simulink model "Heat_Exchanger_v2"  (R2020b)
settings: Solver=ode4  StartTime=0.0  StopTime=1000.0  FixedStep=0.01  RelTol=1e-3
values from neighbouring files (symbols this model uses):
  At = nt .* 2 .* pi .* D_t .* dL    [parat_heat_exchanger.m]
  C_w = 490    [parat_heat_exchanger.m]
  Cp_c = 4005    [parat_heat_exchanger.m]
  Cp_h = 4187    [parat_heat_exchanger.m]
  dt = 0.01    [parat_heat_exchanger.m]
  HTC_ref = 350    [parat_heat_exchanger.m]
  m_ref = 3.5    [parat_heat_exchanger.m]
  mass_c = density_c * Ac * dL    [parat_heat_exchanger.m]
  mass_h = density_h * Ah * dL    [parat_heat_exchanger.m]
  mass_w = density_w * Aw * dL    [parat_heat_exchanger.m]
  mh_start = 2.5    [parat_heat_exchanger.m]
  N = 100    [parat_heat_exchanger.m]
  Tcin = 289    [parat_heat_exchanger.m]
  Tenv = 295    [parat_heat_exchanger.m]
  Thin = 363    [parat_heat_exchanger.m]
  Tref = 348    [parat_heat_exchanger.m]
undefined symbols (not defined in the file or in its folder): Tc_init, Th_init, Tw_init
libraries: pid_lib x1
settings Model: Creator=kzlsahin  LastModifiedBy=kzlsahin

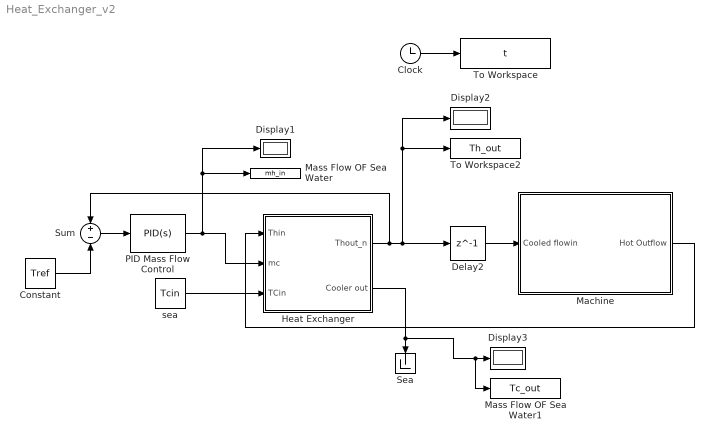
== system Heat_Exchanger_v2 ==
  Clock : Clock
  Constant : Constant  Value=Tref
  Delay2 : Delay  DelayLength=1  InitialCondition=Tenv
  Display1 : Display
  Display2 : Display
  Display3 : Display
  Heat Exchanger : Subsystem
      mask Display: image('/home/kzlsahin/Documents/yüksek lisans/MTME/ödev/iconHXtrans.jpeg'); % Use "Edit Image" on toolstrip to change.
  Machine : Subsystem
  Mass Flow OF Sea Water : ToWorkspace  VariableName=mh_in  SampleTime=-1
  Mass Flow OF Sea Water1 : ToWorkspace  VariableName=Tc_out  SampleTime=-1
  PID Mass Flow Control : pid_lib/PID Controller  Controller=PID  Form=Parallel  TimeDomain=Continuous-time  UseExternalTs=on  SampleTime=-1  IntegratorMethod=Forward Euler  FilterMethod=Forward Euler  ControllerParametersSource=internal  P=1  I=1  D=1  UseFilter=on  N=100  TunerSelectOption=Transfer Function Based (PID Tuner App)  InitialConditionSource=internal  InitialConditionForIntegrator=0  InitialConditionForFilter=0  DifferentiatorICPrevScaledInput=0  ExternalReset=none  TrackingMode=off  Kt=1  LimitOutput=on  SatLimitsSource=internal  UpperSaturationLimit=10  LowerSaturationLimit=0.5  LinearizeAsGain=on  AntiWindupMode=none  Kb=1  POutMin=[]  POutMax=[]  IOutMin=[]  IOutMax=[]  DOutMin=[]  DOutMax=[]  NOutMin=[]  NOutMax=[]  SumOutMin=[]  SumOutMax=[]  SaturationOutMin=[]  SaturationOutMax=[]  PParamMin=[]  PParamMax=[]  IParamMin=[]  IParamMax=[]  DParamMin=[]  DParamMax=[]  NParamMin=[]  NParamMax=[]  KbParamMin=[]  KbParamMax=[]  KtParamMin=[]  KtParamMax=[]  KbOutMin=[]  KbOutMax=[]  KtOutMin=[]  KtOutMax=[]  IntegratorOutMin=[]  IntegratorOutMax=[]  FilterOutMin=[]  FilterOutMax=[]  SumI1OutMin=[]  SumI1OutMax=[]  SumI2OutMin=[]  SumI2OutMax=[]  SumI3OutMin=[]  SumI3OutMax=[]  SumI4OutMin=[]  SumI4OutMax=[]  SumDOutMin=[]  SumDOutMax=[]  DifferentiatorOutMin=[]  DifferentiatorOutMax=[]  FilterDiffOutCoefMin=[]  FilterDiffOutCoefMax=[]  ReciprocalOutMin=[]  ReciprocalOutMax=[]  SumDenOutMin=[]  SumDenOutMax=[]  SumNumOutMin=[]  SumNumOutMax=[]  DivideOutMin=[]  DivideOutMax=[]  UdiffTsProdOutMin=[]  UdiffTsProdOutMax=[]  NTsProdOutMin=[]  NTsProdOutMax=[]  UintegralTsProdOutMin=[]  UintegralTsProdOutMax=[]  UngainTsProdOutMin=[]  UngainTsProdOutMax=[]  IntegratorContinuousStateAttributes=''  IntegratorStateMustResolveToSignalObject=off  IntegratorRTWStateStorageClass=Auto  FilterContinuousStateAttributes=''  FilterStateMustResolveToSignalObject=off  FilterRTWStateStorageClass=Auto  ParallelPVariant=InternalParameters  IdealPVariant=Disabled  IVariant=InternalParameters  DVariant=InternalParameters  IntegratorVariant=Continuous  SatVariant=Enabled  AWVariant=Passthrough  PCopyVariant=Disabled  TRVariant=Disabled  FdbkBlocksVariant=Forward  IdealPFdbkVariant=Disabled  SatFdbkVariant=Disabled  DerivativeFilterVariant=ContFilter  NVariant=InternalParameters  NCopyVariant=Disabled  FilterICVariant=InternalICsFilter  IntegratorICVariant=InternalICs  ExternalResetVariant=Disabled  TRSumVariant=Passthrough  SumFdbkVariant=Disabled  SumVariant=Sum_PID  TsampFilterVariant=InternalTs  TsampNgainVariant=Passthrough  TsampIntegralVariant=Passthrough  ExternalSaturationOutDataTypeStr=Inherit: Same as second input
  Sea : Terminator
  Sum : Sum  Inputs=+-
  To Workspace : ToWorkspace  VariableName=t  SampleTime=-1
  To Workspace2 : ToWorkspace  VariableName=Th_out  SampleTime=-1
  sea : Constant  Value=Tcin
  wires:
  Sum/1 -> PID Mass Flow Control/1
  Machine/1(Hot Outflow) -> Heat Exchanger/1(Thin)
  Clock/1 -> To Workspace/1
  Heat Exchanger/1(Thout_n) -> Display2/1, To Workspace2/1, Delay2/1, Sum/1
  Delay2/1 -> Machine/1(Cooled flowin)
  Heat Exchanger/2(Cooler out) -> Mass Flow OF Sea Water1/1, Display3/1, Sea/1
  sea/1 -> Heat Exchanger/3(TCin)
  PID Mass Flow Control/1 -> Heat Exchanger/2(mc), Display1/1, Mass Flow OF Sea Water/1
  Constant/1 -> Sum/2

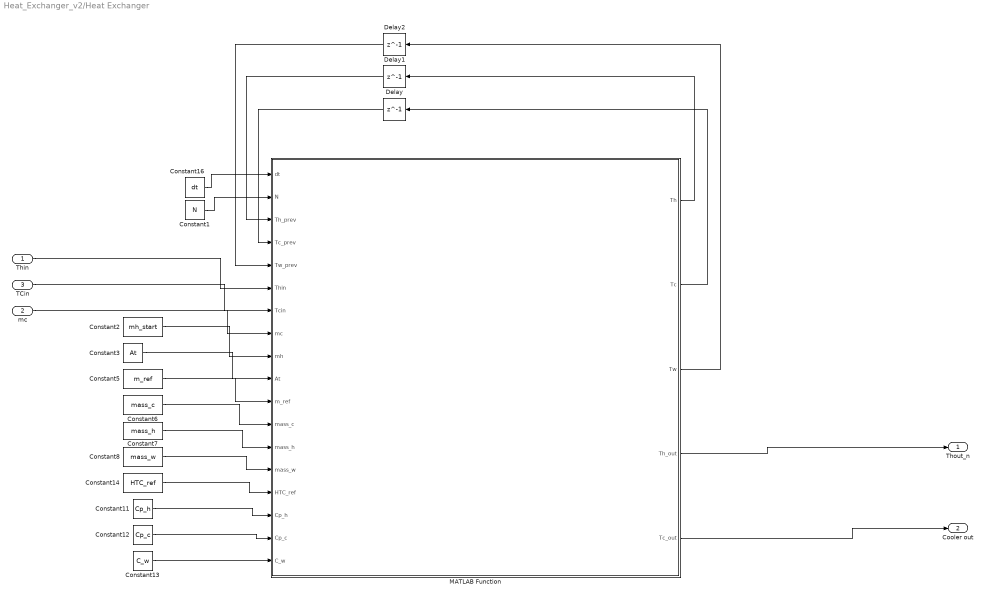
== system Heat_Exchanger_v2/Heat Exchanger ==
  Thin : Inport
  mc : Inport  Port=2
  TCin : Inport  Port=3
  Constant1 : Constant  Value=N
  Constant11 : Constant  Value=Cp_h
  Constant12 : Constant  Value=Cp_c
  Constant13 : Constant  Value=C_w
  Constant14 : Constant  Value=HTC_ref
  Constant16 : Constant  Value=dt
  Constant2 : Constant  Value=mh_start
  Constant3 : Constant  Value=At
  Constant5 : Constant  Value=m_ref
  Constant6 : Constant  Value=mass_c
  Constant7 : Constant  Value=mass_h
  Constant8 : Constant  Value=mass_w
  Delay : Delay  DelayLength=1  InitialCondition=Tc_init
  Delay1 : Delay  DelayLength=1  InitialCondition=Th_init
  Delay2 : Delay  DelayLength=1  InitialCondition=Tw_init
  MATLAB Function : MATLAB Function  TreatAsAtomicUnit=on
  Thout_n : Outport
  Cooler out : Outport  Port=2
  wires:
  MATLAB Function/4(Th_out) -> Thout_n/1
  Thin/1 -> MATLAB Function/6(Thin)
  mc/1 -> MATLAB Function/8(mc)
  TCin/1 -> MATLAB Function/7(Tcin)
  MATLAB Function/5(Tc_out) -> Cooler out/1
  Constant8/1 -> MATLAB Function/14(mass_w)
  Constant7/1 -> MATLAB Function/13(mass_h)
  Constant6/1 -> MATLAB Function/12(mass_c)
  Constant5/1 -> MATLAB Function/11(m_ref)
  Constant3/1 -> MATLAB Function/10(At)
  MATLAB Function/1(Th) -> Delay1/1
  Delay1/1 -> MATLAB Function/3(Th_prev)
  MATLAB Function/2(Tc) -> Delay/1
  Delay/1 -> MATLAB Function/4(Tc_prev)
  Constant11/1 -> MATLAB Function/16(Cp_h)
  Constant12/1 -> MATLAB Function/17(Cp_c)
  Constant13/1 -> MATLAB Function/18(C_w)
  MATLAB Function/3(Tw) -> Delay2/1
  Delay2/1 -> MATLAB Function/5(Tw_prev)
  Constant16/1 -> MATLAB Function/1(dt)
  Constant14/1 -> MATLAB Function/15(HTC_ref)
  Constant1/1 -> MATLAB Function/2(N)
  Constant2/1 -> MATLAB Function/9(mh)

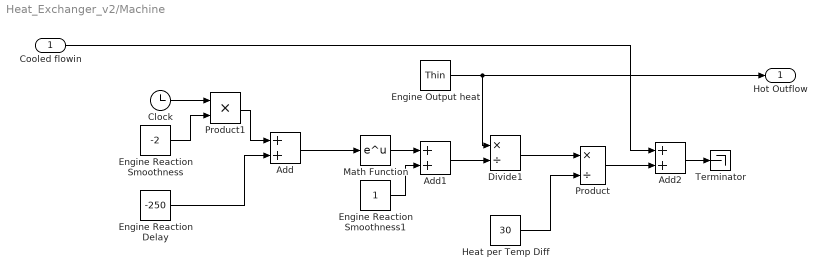
== system Heat_Exchanger_v2/Machine ==
  Cooled flowin : Inport
  Add : Sum
  Add1 : Sum
  Add2 : Sum
  Clock : Clock
  Divide1 : Product  Inputs=*/
  Engine Output heat : Constant  Value=Thin
  Engine Reaction Delay : Constant  Value=-250
  Engine Reaction Smoothness : Constant  Value=-2
  Engine Reaction Smoothness1 : Constant
  Heat per Temp Diff : Constant  Value=30
  Math Function : Math  SaturateOnIntegerOverflow=on
  Product : Product  Inputs=*/
  Product1 : Product
  Terminator : Terminator
  Hot Outflow : Outport
  wires:
  Clock/1 -> Product1/1
  Add/1 -> Math Function/1
  Product1/1 -> Add/1
  Engine Reaction Smoothness/1 -> Product1/2
  Engine Reaction Delay/1 -> Add/2
  Math Function/1 -> Add1/1
  Engine Reaction Smoothness1/1 -> Add1/2
  Engine Output heat/1 -> Divide1/1, Hot Outflow/1
  Add1/1 -> Divide1/2
  Divide1/1 -> Product/1
  Heat per Temp Diff/1 -> Product/2
  Product/1 -> Add2/2
  Add2/1 -> Terminator/1
  Cooled flowin/1 -> Add2/1

== matlab function Heat_Exchanger_v2/Heat Exchanger/MATLAB Function ==
  data: dt input; N input; Th output; Tc output; Tw output; Th_prev input; Tc_prev input; Tw_prev input; Thin input; Tcin input; mc input; mh input; At input; m_ref input; mass_c input; mass_h input; mass_w input; Th_out output; HTC_ref input; Tc_out output; Cp_h input; Cp_c input; C_w input
function [Th, Tc, Tw,Th_out, Tc_out] = fcn(dt,N,Th_prev, Tc_prev,Tw_prev, Thin,Tcin,mc,mh,At,m_ref,mass_c,mass_h,mass_w,HTC_ref,Cp_h,Cp_c, C_w)
%Counter flow heat exchanger with tubes inside circular section

%this function is suitable for a heat exchanger system that the cold fluid
%flows through shell and the hot fluid flows through tubes.
%assumptions are made for this simulation:
% - temperatures at the entering points are assumed to be fixed
% - becouse of the counter flow, the temperature spread is assumed to be
% linear during the length of the tubes
% author Mustafa ŞENTÜRK

HTCh = HTC_ref * (mh / m_ref)^0.6;
HTCc = HTC_ref * (mc / m_ref)^0.6;

Tw = zeros(size(Tw_prev));
Th = zeros(size(Th_prev));
Tc = zeros(size(Tc_prev));

Th(1) = Thin;
Tc(N+1) = Tcin;

% n is the index of the segment
for n=1:1:N
    i = n + 1; % indexes of Th as Th(1) is in fact Th(0)
    Tw(n) = Tw_prev(n) + ( HTCh.*At.*(Th_prev(n) - Tw_prev(n)) + HTCc.*At.*(Tc_prev(n) - Tw_prev(n))) .* dt / (mass_w .* C_w);
    Th(i) = Th_prev(i) + (mh .* Cp_h .* (Th_prev(i-1) - Th_prev(i)) + HTCh.*At.*(Tw_prev(n) - Th_prev(i))) .* dt / (mass_h .* Cp_h);
    Tc(n) = Tc_prev(n) + (mc .* Cp_c .* (Tc_prev(n+1) - Tc_prev(n)) + HTCc.*At.*(Tw_prev(n) - Tc_prev(n))) .* dt / (mass_c .* Cp_c);

end

Th_out = Th(N+1);
Tc_out = Tc(1);
